simulink model "copper_solvent_extraction_model_simulink"  (R2021a)
settings: Solver=ode14x  StartTime=0.0  StopTime=simulation_time  FixedStep=step_time  RelTol=1e-3
undefined symbols (not defined in the file): C1_aq_ss, C1_el_ss, C1_org_ss, C2_aq_ss, C2_org_ss, C3_aq_ss, C3_org_ss, C4_org_ss, C_aq_max, C_org_max, cLE_ss, cPLS_ss, EXTERNAL_VARIABLES_STEADY_STATE, fLE_max, fLO_max, fPLSP_ss, fPLSS_ss, I_FB1, I_FB2, K_eq_ext, K_eq_str, K_ff_FF1, K_ff_FF2, K_ff_FF3, K_ff_FF4, K_mass_1, K_mass_2, K_mass_3, K_mass_4, Kb_FB1, Kb_FB2, Kc_FB1, Kc_FB2, LOWPASS_FILTER_TUNING, seed_c_BO, seed_c_LE, seed_c_LO, seed_c_PLS, seed_c_RaffP, seed_c_RaffS, seed_c_RE, seed_f_LE, seed_f_LO, seed_f_PLSP, seed_f_PLSS, sigma_c_BO, sigma_c_LE, sigma_c_LO, sigma_c_PLS, sigma_c_RaffP, sigma_c_RaffS, sigma_c_RE, sigma_f_LE, sigma_f_LO, sigma_f_PLSP, sigma_f_PLSS, step_time, t1, t2, t3 ... (+43)
libraries: cstblocks x4, pid_lib x2
(part 3 of 3)

== stateflow chart copper_solvent_extraction_model_simulink/Valve LE/Variant Subsystem/Valve LE State Normal/Valve LE Finite State Machine Normal ==
  state Normal
    entry, during:
    valve_LE_state = 0;
    v_LE_is_not_stuck = 1;
  state Stuck
    entry:
    valve_LE_state = 1;
    during:
    valve_LE_state = 1;
    v_LE_is_not_stuck = 0;
  state Stiction
    entry:
    valve_LE_state = 2;
    valve_LE_stiction_v_initial = v_LE_valve_previous;
    valve_LE_stiction_start_time = simulation_time;
    during:
    valve_LE_state = 2;
  (default) -> Normal
  data: valve_LE_state output; simulation_time input; v_LE_is_not_stuck output; valve_LE_fault_start_time parameter; valve_LE_fault_stop_time parameter; valve_LE_stiction_v_initial output; v_LE_valve_previous input; valve_LE_stiction_start_time output

== stateflow chart copper_solvent_extraction_model_simulink/Valve LE/Variant Subsystem/Valve LE State Stiction/Valve LE Finite State Machine Stiction ==
  state Normal
    entry, during:
    valve_LE_state = 0;
    v_LE_is_not_stuck = 1;
  state Stuck
    entry:
    valve_LE_state = 1;
    during:
    valve_LE_state = 1;
    v_LE_is_not_stuck = 0;
  state Stiction
    entry:
    valve_LE_state = 2;
    valve_LE_stiction_v_initial = v_LE_valve_previous;
    valve_LE_stiction_start_time = simulation_time;
    during:
    valve_LE_state = 2;
  (default) -> Normal
  Normal -> Stiction : [simulation_time == valve_LE_fault_start_time]
  Stiction -> Normal : [simulation_time == valve_LE_fault_stop_time]
  data: valve_LE_state output; simulation_time input; v_LE_is_not_stuck output; valve_LE_fault_start_time parameter; valve_LE_fault_stop_time parameter; valve_LE_stiction_v_initial output; v_LE_valve_previous input; valve_LE_stiction_start_time output

== stateflow chart copper_solvent_extraction_model_simulink/Valve LE/Variant Subsystem/Valve LE State Stuck/Valve LE Finite State Machine Stuck ==
  state Normal
    entry, during:
    valve_LE_state = 0;
    v_LE_is_not_stuck = 1;
  state Stuck
    entry:
    valve_LE_state = 1;
    during:
    valve_LE_state = 1;
    v_LE_is_not_stuck = 0;
  state Stiction
    entry:
    valve_LE_state = 2;
    valve_LE_stiction_v_initial = v_LE_valve_previous;
    valve_LE_stiction_start_time = simulation_time;
    during:
    valve_LE_state = 2;
  (default) -> Normal
  Normal -> Stuck : [simulation_time == valve_LE_fault_start_time]
  Stuck -> Normal : [simulation_time == valve_LE_fault_stop_time]
  data: valve_LE_state output; simulation_time input; v_LE_is_not_stuck output; valve_LE_fault_start_time parameter; valve_LE_fault_stop_time parameter; valve_LE_stiction_v_initial output; v_LE_valve_previous input; valve_LE_stiction_start_time output

== matlab function copper_solvent_extraction_model_simulink/Simulation Scopes/MATLAB Function ==
  data: valve_LO_state input; simulation_process_state output; valve_LE_state input
function simulation_process_state = fcn(valve_LO_state, valve_LE_state)

    % Initial value
    simulation_process_state = 0;    

    % Process state 0
    if((valve_LO_state == 0) && (valve_LE_state == 0))
        simulation_process_state = 0;
    end
    
    % Process state 1
    if((valve_LO_state == 1) && (valve_LE_state == 0))
        simulation_process_state = 1;
    end
    
    % Process state 2
    if((valve_LO_state == 2) && (valve_LE_state == 0))
        simulation_process_state = 2;
    end
    
    % Process state 3
    if((valve_LO_state == 0) && (valve_LE_state == 1))
        simulation_process_state = 3;
    end
    
    % Process state 4
    if((valve_LO_state == 0) && (valve_LE_state == 2))
        simulation_process_state = 4;
    end
    
    % Process state 5
    if((valve_LO_state == 1) && (valve_LE_state == 1))
        simulation_process_state = 5;
    end
    
    % Process state 6
    if((valve_LO_state == 1) && (valve_LE_state == 2))
        simulation_process_state = 6;
    end
    
    % Process state 7
    if((valve_LO_state == 2) && (valve_LE_state == 1))
        simulation_process_state = 7;
    end
    
    % Process state 8
    if((valve_LO_state == 2) && (valve_LE_state == 2))
        simulation_process_state = 8;
    end
    
end

== matlab function copper_solvent_extraction_model_simulink/Extraction E2/Mixer E2/Mixer E2 MATLAB Function ==
  data: fPLSS input; C3_aq_delay input; fLO input; C1_org_delay input; C2_org input; C2_org_equilibrium output; C2_aq input; K_mass_2 parameter; V2 parameter; dC2_org_dt output; dC2_aq_dt output; C_org_max parameter; K_eq_ext parameter
function [C2_org_equilibrium, dC2_org_dt, dC2_aq_dt] = fcn(fPLSS, C3_aq_delay, fLO, C1_org_delay, C2_org, C2_aq, K_mass_2, V2, C_org_max, K_eq_ext)

% Extraction unit E2's Mixer

% The parameters are imported from the workspace, therefore run the
% simulation from the /process_model/copper_solvent_extraction_model.mlx
% live script.

% Dynamic equilibrium
C2_org_equilibrium = (C_org_max * C2_aq)./((1./K_eq_ext) + C2_aq);

% Mass balances 
dC2_org_dt = (fLO/V2)*(C1_org_delay - C2_org) + K_mass_2*(C2_org_equilibrium - C2_org);
dC2_aq_dt  = (fPLSS/V2)*(C3_aq_delay - C2_aq) - K_mass_2*(C2_org_equilibrium - C2_org);

end

== stateflow chart copper_solvent_extraction_model_simulink/Valve LO/Variant Subsystem/Valve LO State Normal/Valve LO Finite State Machine Normal ==
  state Normal
    entry, during:
    valve_LO_state = 0;
    v_LO_is_not_stuck = 1;
  state Stuck
    entry:
    valve_LO_state = 1;
    during:
    valve_LO_state = 1;
    v_LO_is_not_stuck = 0;
  state Stiction
    entry:
    valve_LO_state = 2;
    valve_LO_stiction_v_initial = v_LO_valve_previous;
    valve_LO_stiction_start_time = simulation_time;
    during:
    valve_LO_state = 2;
  (default) -> Normal
  data: valve_LO_state output; simulation_time input; v_LO_is_not_stuck output; valve_LO_fault_start_time parameter; valve_LO_fault_stop_time parameter; valve_LO_stiction_v_initial output; v_LO_valve_previous input; valve_LO_stiction_start_time output

== matlab function copper_solvent_extraction_model_simulink/Extraction E3/Mixer E3/Mixer E3 MATLAB Function ==
  data: fPLSS input; cPLS input; C3_org_equilibrium output; fLO input; C2_org_delay input; C3_org input; C3_aq input; K_mass_3 parameter; V3 parameter; dC3_org_dt output; dC3_aq_dt output; C_org_max parameter; K_eq_ext parameter
function [C3_org_equilibrium, dC3_org_dt, dC3_aq_dt] = fcn(fPLSS, cPLS, fLO, C2_org_delay, C3_org, C3_aq, K_mass_3, V3, C_org_max, K_eq_ext)

% Extraction unit E3's Mixer

% The parameters are imported from the workspace, therefore run the
% simulation from the /process_model/copper_solvent_extraction_model.mlx
% live script.

% Dynamic equilibrium
C3_org_equilibrium = (C_org_max * C3_aq)./((1./K_eq_ext) + C3_aq);

% Mass balances 
dC3_org_dt = (fLO/V3)*(C2_org_delay - C3_org) + K_mass_3*(C3_org_equilibrium - C3_org); 
dC3_aq_dt  = (fPLSS/V3)*(cPLS - C3_aq)        - K_mass_3*(C3_org_equilibrium - C3_org);

end
